simulink model "mqtt_simulink_24b"  (R2024b)
settings: Solver=ode5  StartTime=0.0  StopTime=inf  RelTol=1e-3
PreLoadFcn:
  | modellSti = fileparts(which(bdroot));
  | addpath(genpath(fullfile(modellSti, 'mqtt')));
  | addpath(genpath('mqtt'));
libraries: read_b x4, send_b x3, init x1
settings Model: Creator=adriaeik  LastModifiedBy=eikel
settings HardwareCC: ProdBitPerLong=64  ProdHWDeviceType=Intel->x86-64 (Linux 64)
settings RTWCC: Description=Simulink Desktop Real-Time  SystemTargetFile=sldrt.tlc  TemplateMakefile=sldrt.tmf  TargetLang=C++  RTWCompilerOptimization=on
settings CodeAppCC: MaxIdLength=95
settings SimulinkDesktopRealTimeCC: TargetLibSuffix=_sldrt.a  TargetPreCompLibLocation=C:\Program Files\MATLAB\R2024a\toolbox\sldrt\lib\win64  TargetLangStandard=C++11 (ISO)  CCListing=on  RebuildAll=on

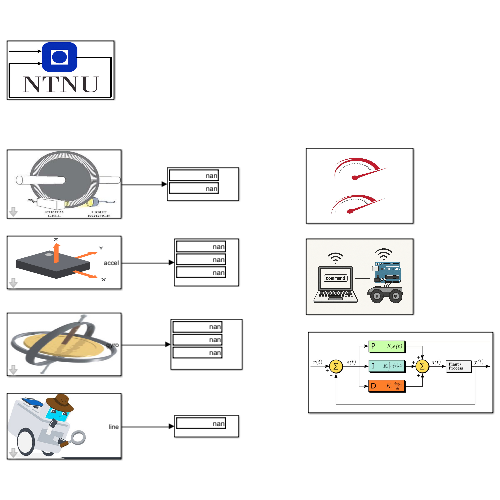
[thumbnail: Simulink's stored preview of the top-level diagram]
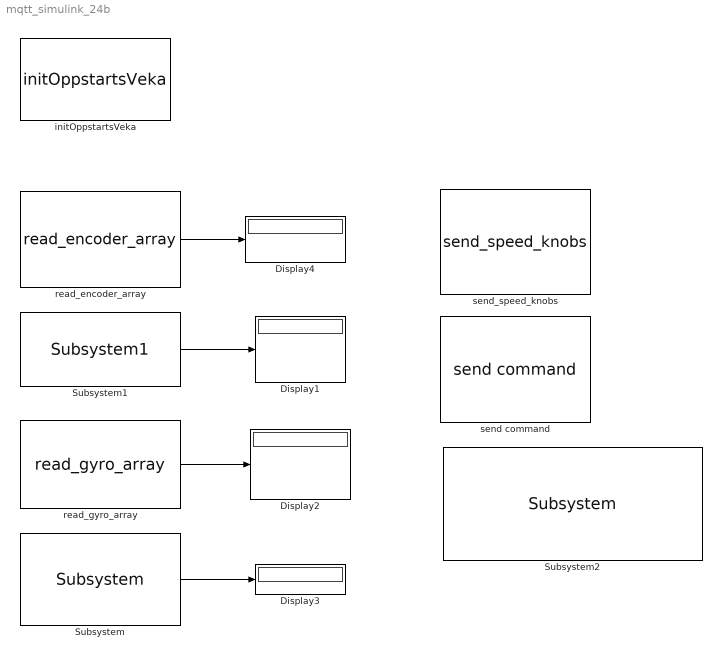
== system mqtt_simulink_24b ==
  Display{1..4} (4 alike) : Display
  Subsystem : read_b/Subsystem
  Subsystem1 : read_b/Subsystem1
  Subsystem2 : send_b/Subsystem  kp=0  ki=0  kd=0
  initOppstartsVeka : init/initOppstartsVeka  carID=14
  read_encoder_array : read_b/read_encoder_array
  read_gyro_array : read_b/read_gyro_array
  send command : send_b/send command  cmd=start
  send_speed_knobs : send_b/send_speed_knobs  left=264.0  right=184.0
  wires:
  Subsystem1/1 -> Display1/1
  read_gyro_array/1 -> Display2/1
  Subsystem/1 -> Display3/1
  read_encoder_array/1 -> Display4/1
